simulink model "Compensator_test"  (R2014a)
settings: Solver=ode45  StartTime=0.0  StopTime=10.0  FixedStep=dt/10  MaxStep=10*dt  MinStep=dt/1000  RelTol=1e-5
values from neighbouring files (symbols this model uses):
  amp_cl = diag(diag(1./squeeze(real(ystp_cl(end,:,:)))))    [forceControMatl_linearModel.m]    (also in simulation_w_compensator.m = eye(3))
undefined symbols (not defined in the file or in its folder): Atf, Dtf
libraries: cstblocks x12
settings Model: Creator=Ron  LastModifiedBy=Ron
settings SolverCC: InitialStep=dt

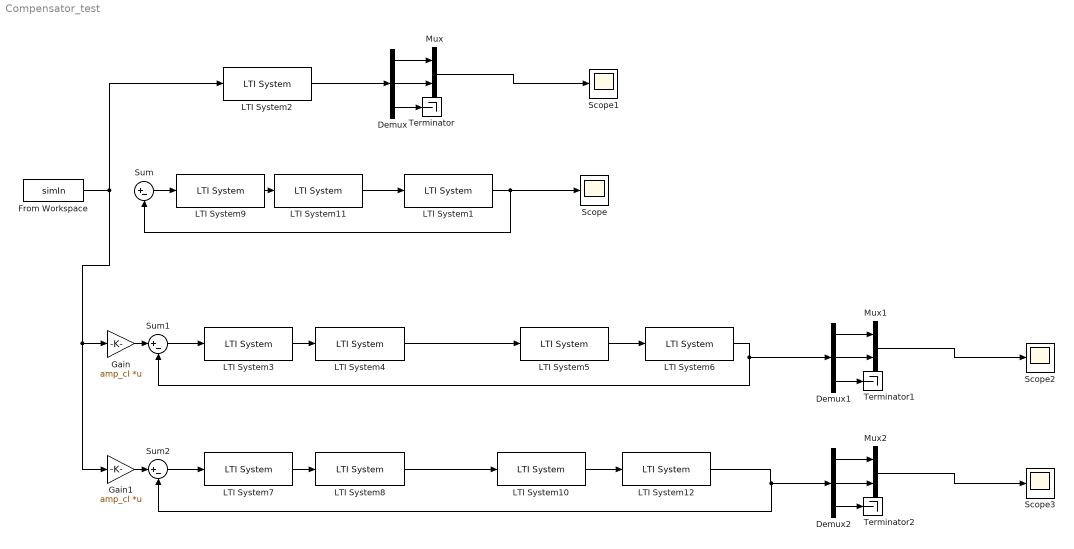
== system Compensator_test ==
  Demux : Demux  Outputs=3
  Demux1 : Demux  Outputs=3
  Demux2 : Demux  Outputs=3
  From Workspace : FromWorkspace  VariableName=simIn  SampleTime=0
  Gain : Gain  Gain=amp_cl  Multiplication=Matrix(K*u)
  Gain1 : Gain  Gain=amp_cl  Multiplication=Matrix(K*u)
  LTI System1 : cstblocks/LTI System  sys=G_ol  IC=[0]
  LTI System10 : cstblocks/LTI System  sys=Dtf^-1  IC=[0]
  LTI System11 : cstblocks/LTI System  sys=Atf^-1  IC=[0]
  LTI System12 : cstblocks/LTI System  sys=Ntf  IC=[0]
  LTI System2 : cstblocks/LTI System  sys=G_cl  IC=[0]
  LTI System3 : cstblocks/LTI System  sys=Btf  IC=[0]
  LTI System4 : cstblocks/LTI System  sys=Atf^-1  IC=[0]
  LTI System5 : cstblocks/LTI System  sys=Dtf^-1  IC=[0]
  LTI System6 : cstblocks/LTI System  sys=Ntf  IC=[0]
  LTI System7 : cstblocks/LTI System  sys=Btf  IC=[0]
  LTI System8 : cstblocks/LTI System  sys=Atf^-1  IC=[0]
  LTI System9 : cstblocks/LTI System  sys=Btf  IC=[0]
  Mux : Mux  Inputs=2
  Mux1 : Mux  Inputs=2
  Mux2 : Mux  Inputs=2
  Scope{,1..3} (4 alike) : Scope
      Scope settings: YMin=-9e+54  YMax=-9676.64
      Scope1 settings: YMin=0.03  YMax=0.11
      Scope2 settings: SaveName=ScopeData2
      Scope3 settings: SaveName=ScopeData3
  Sum : Sum  Inputs=|+-
  Sum1 : Sum  Inputs=|+-
  Sum2 : Sum  Inputs=|+-
  Terminator : Terminator
  Terminator1 : Terminator
  Terminator2 : Terminator
  wires:
  LTI System1/1 -> Scope/1, Sum/2
  LTI System5/1 -> LTI System6/1
  Gain/1 -> Sum1/1
  Demux/1 -> Mux/1
  Demux/2 -> Mux/2
  Demux/3 -> Terminator/1
  LTI System2/1 -> Demux/1
  Mux/1 -> Scope1/1
  Demux1/1 -> Mux1/1
  Demux1/2 -> Mux1/2
  Demux1/3 -> Terminator1/1
  LTI System6/1 -> Demux1/1, Sum1/2
  Mux1/1 -> Scope2/1
  LTI System4/1 -> LTI System5/1
  LTI System3/1 -> LTI System4/1
  Sum1/1 -> LTI System3/1
  LTI System9/1 -> LTI System11/1
  Sum/1 -> LTI System9/1
  LTI System11/1 -> LTI System1/1
  Gain1/1 -> Sum2/1
  Demux2/1 -> Mux2/1
  Demux2/2 -> Mux2/2
  Demux2/3 -> Terminator2/1
  Mux2/1 -> Scope3/1
  From Workspace/1 -> LTI System2/1, Gain1/1, Gain/1
  LTI System7/1 -> LTI System8/1
  Sum2/1 -> LTI System7/1
  LTI System10/1 -> LTI System12/1
  LTI System8/1 -> LTI System10/1
  LTI System12/1 -> Sum2/2, Demux2/1
